simulink model "Induction_machine_qd0model_Turr"  (R2021b)
settings: Solver=FixedStepDiscrete  StartTime=0.0  StopTime=10  FixedStep=Ts  RelTol=1e-3
InitFcn:
  | Ts=1e-5;
  | fe=50;
  | Vrms=230;
undefined symbols (not defined in the file): DiscIntNeverNeededParam
settings Model: Creator=tturr  LastModifiedBy=lecci

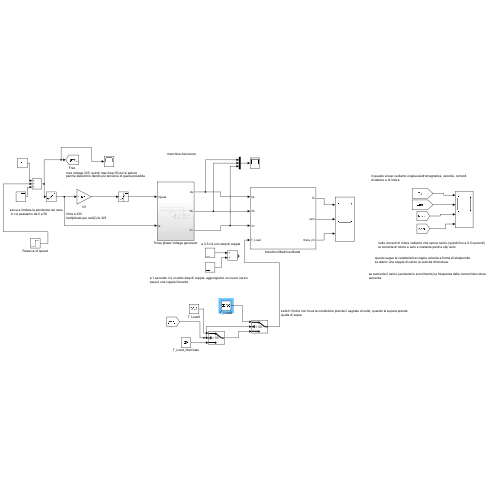
[thumbnail: Simulink's stored preview of the top-level diagram]
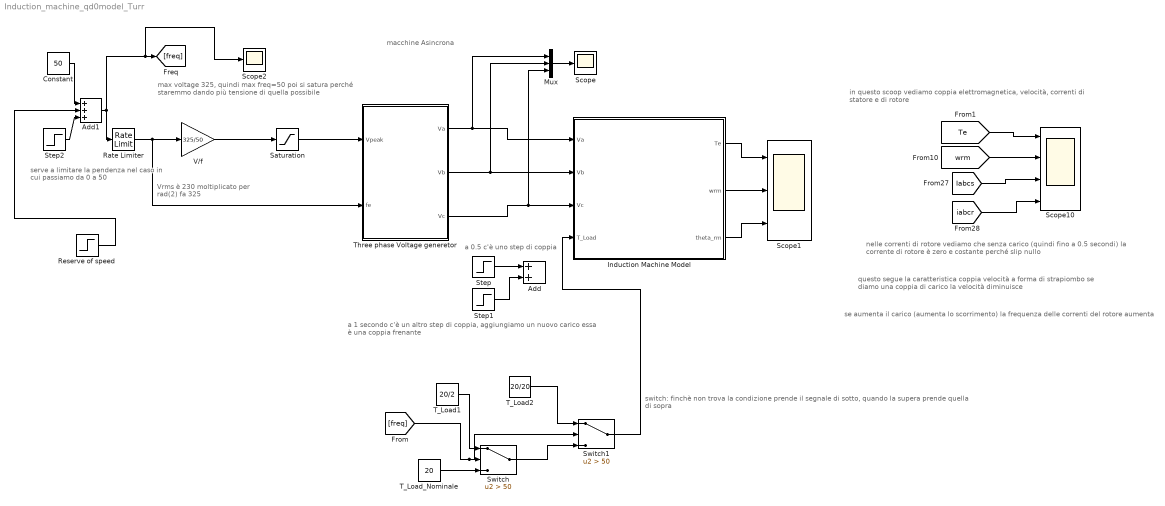
== system Induction_machine_qd0model_Turr ==
  note: switch: finchè non trova la condizione prende il segnale di sotto, quando la supera prende quella di sopra
  note: serve a limitare la pendenza nel caso
      |  in cui passiamo da 0 a 50
  note: max voltage 325, quindi max freq=50 poi si satura
      | perché staremmo dando più tensione di quella possibile
  note: Vrms è 230
      | moltiplicato per rad(2) fa 325
  note: se aumenta il carico (aumenta lo scorrimento) la frequenza delle correnti del rotore aumenta
  note: questo segue la caratteristica coppia velocità a forma di strapiombo
      | se diamo una coppia di carico la velocità diminuisce
  note: macchine Asincrona
  note: nelle correnti di rotore vediamo che senza carico (quindi fino a 0.5 secondi)
      | la corrente di rotore è zero e costante perché slip nullo
  note: in questo scoop vediamo coppia elettromagnetica, velocità, correnti
      | di statore e di rotore
  note: a 1 secondo c'è un altro step di coppia, aggiungiamo un nuovo carico
      | essa è una coppia frenante
  note: a 0.5 c'è uno step di coppia
  Add : Sum
  Add1 : Sum  Inputs=+++
  Constant : Constant  Value=50
  "Induction Machine Model " : Subsystem
  Mux : Mux  Inputs=3
  Rate Limiter : RateLimiter  RisingSlewLimit=50  FallingSlewLimit=-50  SampleTimeMode=inherited
  Reserve of speed : Step  Time=4  After=70  SampleTime=0
  Saturation : Saturate  UpperLimit=325  LowerLimit=-325
  Scope : Scope
  Scope1 : Scope  NumInputPorts=3
  Scope10 : Scope  NumInputPorts=4
  Scope2 : Scope
  Step : Step  Time=0.5  After=20  SampleTime=0
  Step1 : Step  After=20  SampleTime=0
  Step2 : Step  Time=2  After=50  SampleTime=0
  Switch : Switch  Criteria=u2 > Threshold  Threshold=50
  Switch1 : Switch  Criteria=u2 > Threshold  Threshold=50
  T_Load1 : Constant  Value=20/2
  T_Load2 : Constant  Value=20/20
  T_Load_Nominale : Constant  Value=20
  Three phase Voltage generetor : Subsystem
  V/f : Gain  Gain=325/50
  wires:
  Saturation/1 -> Three phase Voltage generetor/1(Vpeak)
  Mux/1 -> Scope/1
  Step/1 -> Add/1
  "Induction Machine Model "/2(wrm) -> Scope1/2
  "Induction Machine Model "/1(Te) -> Scope1/1
  "Induction Machine Model "/3(theta_rm) -> Scope1/3
  [wrm] -> Scope10/2
  [Te] -> Scope10/1
  [Iabcs] -> Scope10/3
  [iabcr] -> Scope10/4
  Step1/1 -> Add/2
  Three phase Voltage generetor/3(Vc) -> Mux/3, "Induction Machine Model "/3(Vc)
  Three phase Voltage generetor/2(Vb) -> Mux/2, "Induction Machine Model "/2(Vb)
  Three phase Voltage generetor/1(Va) -> Mux/1, "Induction Machine Model "/1(Va)
  V/f/1 -> Saturation/1
  Rate Limiter/1 -> Three phase Voltage generetor/2(fe), V/f/1
  Constant/1 -> Add1/1
  Step2/1 -> Add1/3
  Add1/1 -> Scope2/1, [freq], Rate Limiter/1
  T_Load_Nominale/1 -> Switch/3
  [freq] -> Switch1/2, Switch/2
  T_Load1/1 -> Switch/1
  Reserve of speed/1 -> Add1/2
  Switch/1 -> Switch1/3
  T_Load2/1 -> Switch1/1
  Switch1/1 -> "Induction Machine Model "/4(T_Load)

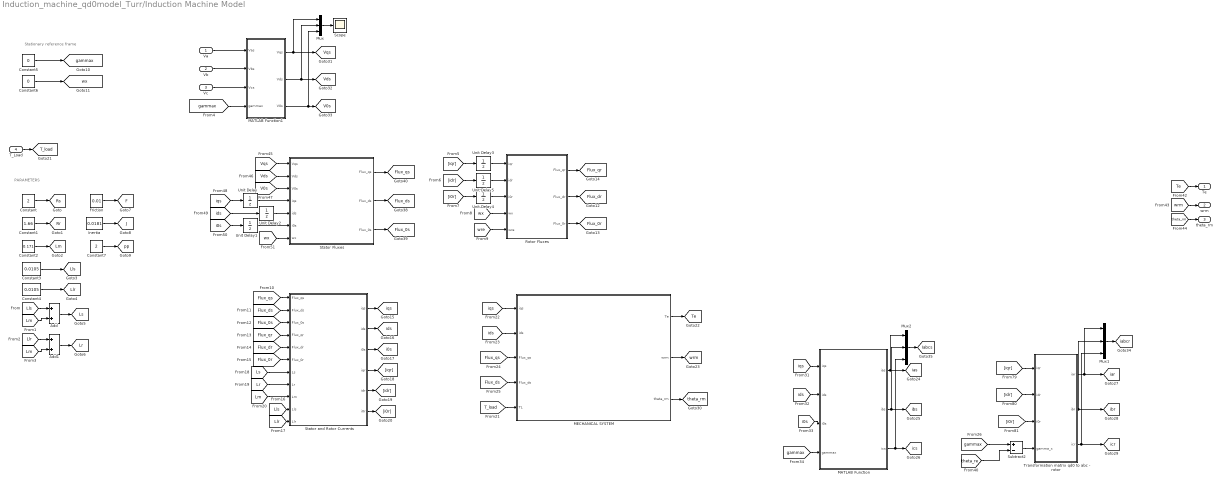
== system Induction_machine_qd0model_Turr/Induction Machine Model  ==
  note: Stationary reference frame
  note: PARAMETERS
  Va : Inport
  Vb : Inport  Port=2
  Vc : Inport  Port=3
  T_Load : Inport  Port=4
  Add : Sum
  Add1 : Sum
  Constant : Constant  Value=2
  Constant1 : Constant  Value=1.66
  Constant2 : Constant  Value=0.171
  Constant3 : Constant  Value=0.0105
  Constant4 : Constant  Value=0.0105
  Constant5 : Constant  Value=0
  Constant6 : Constant  Value=0
  Constant7 : Constant  Value=2
  Friction : Constant  Value=0.01
  Inertia : Constant  Value=0.0181
  MATLAB Function : MATLAB Function  TreatAsAtomicUnit=on
  MATLAB Function1 : MATLAB Function  TreatAsAtomicUnit=on
  MECHANICAL SYSTEM : Subsystem
  Mux : Mux  Inputs=3
  Mux1 : Mux  Inputs=3
  Mux2 : Mux  Inputs=3
  Rotor Fluxes : Subsystem
  Scope : Scope
  Stator Fluxes : Subsystem
  Stator and Rotor Currents : MATLAB Function  TreatAsAtomicUnit=on
  Subtract2 : Sum  Inputs=+-
  Transformation matrix qd0 to abc - rotor : MATLAB Function  TreatAsAtomicUnit=on
  Unit Delay{,1..5} (6 alike) : UnitDelay  SampleTime=-1  HasFrameUpgradeWarning=on
  Te : Outport
  wrm : Outport  Port=2
  theta_rm : Outport  Port=3
  tag scope: F=global, Flux_0r=global, Flux_0s=global, Flux_dr=global, Flux_ds=global, Flux_qr=global, Flux_qs=global, Iabcs=global, J=global, Llr=global, Lls=global, Lm=global, Lr=global, Ls=global, Rr=global, Rs=global, T_load=global, Te=global, V0s=global, Vds=global, Vqs=global, gammax=global, i0s=global, iabcr=global, iar=global, ias=global, ibr=global, ibs=global, icr=global, ics=global, ids=global, iqs=global, pp=global, theta_rm=global, wrm=global, wx=global
  wires:
  Constant/1 -> [Rs]
  Constant1/1 -> [Rr]
  Constant2/1 -> [Lm]
  Constant3/1 -> [Lls]
  Constant4/1 -> [Llr]
  Add/1 -> [Ls]
  [Lls] -> Add/1
  [Lm] -> Add/2
  [Lm] -> Add1/2
  [Llr] -> Add1/1
  Add1/1 -> [Lr]
  Constant7/1 -> [pp]
  Inertia/1 -> [J]
  Friction/1 -> [F]
  Va/1 -> MATLAB Function1/1(Vas)
  Vb/1 -> MATLAB Function1/2(Vbs)
  Vc/1 -> MATLAB Function1/3(Vcs)
  Constant5/1 -> [gammax]
  Constant6/1 -> [wx]
  [gammax] -> MATLAB Function1/4(gammax)
  Mux/1 -> Scope/1
  MATLAB Function1/1(Vqs) -> Mux/1, [Vqs]
  MATLAB Function1/2(Vds) -> [Vds], Mux/2
  MATLAB Function1/3(V0s) -> [V0s], Mux/3
  [Te] -> Te/1
  [wrm] -> wrm/1
  [theta_rm] -> theta_rm/1
  Stator Fluxes/1(Flux_qs) -> [Flux_qs]
  Stator Fluxes/2(Flux_ds) -> [Flux_ds]
  Stator Fluxes/3(Flux_0s) -> [Flux_0s]
  [Vqs] -> Stator Fluxes/1(Vqs)
  [Vds] -> Stator Fluxes/2(Vds)
  [V0s] -> Stator Fluxes/3(V0s)
  [ids] -> Unit Delay2/1
  [i0s] -> Unit Delay1/1
  [wx] -> Stator Fluxes/7(wx)
  [iqs] -> Unit Delay/1
  Unit Delay/1 -> Stator Fluxes/4(iqs)
  Unit Delay1/1 -> Stator Fluxes/6(i0s)
  Unit Delay2/1 -> Stator Fluxes/5(ids)
  [iqr] -> Unit Delay3/1
  [i0r] -> Unit Delay4/1
  [idr] -> Unit Delay5/1
  Unit Delay3/1 -> Rotor Fluxes/1(iqr)
  Unit Delay5/1 -> Rotor Fluxes/2(idr)
  Unit Delay4/1 -> Rotor Fluxes/3(i0r)
  [wx] -> Rotor Fluxes/4(wx)
  [wre] -> Rotor Fluxes/5(wre)
  Rotor Fluxes/1(Flux_qr) -> [Flux_qr]
  Rotor Fluxes/2(Flux_dr) -> [Flux_dr]
  Rotor Fluxes/3(Flux_0r) -> [Flux_0r]
  Stator and Rotor Currents/1(iqs) -> [iqs]
  Stator and Rotor Currents/2(ids) -> [ids]
  Stator and Rotor Currents/3(i0s) -> [i0s]
  Stator and Rotor Currents/4(iqr) -> [iqr]
  Stator and Rotor Currents/5(idr) -> [idr]
  Stator and Rotor Currents/6(i0r) -> [i0r]
  [Flux_qs] -> Stator and Rotor Currents/1(Flux_qs)
  [Flux_ds] -> Stator and Rotor Currents/2(Flux_ds)
  [Flux_0s] -> Stator and Rotor Currents/3(Flux_0s)
  [Flux_qr] -> Stator and Rotor Currents/4(Flux_qr)
  [Flux_dr] -> Stator and Rotor Currents/5(Flux_dr)
  [Flux_0r] -> Stator and Rotor Currents/6(Flux_0r)
  [Ls] -> Stator and Rotor Currents/7(Ls)
  [Lr] -> Stator and Rotor Currents/8(Lr)
  [Lm] -> Stator and Rotor Currents/9(Lm)
  [Lls] -> Stator and Rotor Currents/10(Lls)
  [Llr] -> Stator and Rotor Currents/11(Llr)
  Transformation matrix qd0 to abc - rotor/3(icr) -> Mux1/3, [icr]
  [idr] -> Transformation matrix qd0 to abc - rotor/2(idr)
  [i0r] -> Transformation matrix qd0 to abc - rotor/3(i0r)
  [ids] -> MATLAB Function/2(ids)
  MATLAB Function/3(ics) -> Mux2/3, [ics]
  Transformation matrix qd0 to abc - rotor/1(iar) -> Mux1/1, [iar]
  MATLAB Function/1(ias) -> Mux2/1, [ias]
  [theta_re] -> Subtract2/2
  [iqr] -> Transformation matrix qd0 to abc - rotor/1(iqr)
  Subtract2/1 -> Transformation matrix qd0 to abc - rotor/4(gamma_x)
  MATLAB Function/2(ibs) -> Mux2/2, [ibs]
  [gammax] -> MATLAB Function/4(gammax)
  [iqs] -> MATLAB Function/1(iqs)
  [i0s] -> MATLAB Function/3(i0s)
  [gammax] -> Subtract2/1
  T_Load/1 -> [T_load]
  [T_load] -> MECHANICAL SYSTEM/5(TL)
  [iqs] -> MECHANICAL SYSTEM/1(iqs)
  [ids] -> MECHANICAL SYSTEM/2(ids)
  [Flux_ds] -> MECHANICAL SYSTEM/4(Flux_ds)
  [Flux_qs] -> MECHANICAL SYSTEM/3(Flux_qs)
  MECHANICAL SYSTEM/1(Te) -> [Te]
  MECHANICAL SYSTEM/2(wrm) -> [wrm]
  MECHANICAL SYSTEM/3(theta_rm) -> [theta_rm]
  Transformation matrix qd0 to abc - rotor/2(ibr) -> Mux1/2, [ibr]
  Mux1/1 -> [iabcr]
  Mux2/1 -> [Iabcs]

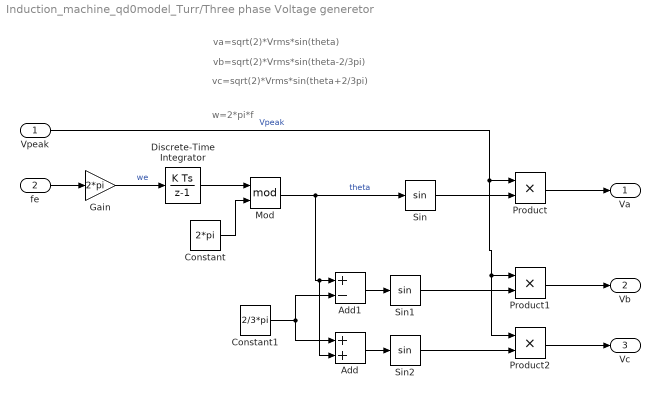
== system Induction_machine_qd0model_Turr/Three phase Voltage generetor ==
  note: w=2*pi*f
  note: va=sqrt(2)*Vrms*sin(theta)
  note: vb=sqrt(2)*Vrms*sin(theta-2/3pi)
  note: vc=sqrt(2)*Vrms*sin(theta+2/3pi)
  Vpeak : Inport
  fe : Inport  Port=2
  Add : Sum
  Add1 : Sum  Inputs=+-
  Constant : Constant  Value=2*pi
  Constant1 : Constant  Value=2/3*pi
  Discrete-Time Integrator : DiscreteIntegrator  SampleTime=-1  ICPrevOutput=DiscIntNeverNeededParam  ICPrevScaledInput=DiscIntNeverNeededParam
  Gain : Gain  Gain=2*pi
  Mod : Math  Operator=mod  SaturateOnIntegerOverflow=on
  Product : Product
  Product1 : Product
  Product2 : Product
  Sin : Trigonometry
  Sin1 : Trigonometry
  Sin2 : Trigonometry
  Va : Outport
  Vb : Outport  Port=2
  Vc : Outport  Port=3
  wires:
  fe/1 -> Gain/1
  Gain/1 -> Discrete-Time Integrator/1  "we"
  Discrete-Time Integrator/1 -> Mod/1
  Constant/1 -> Mod/2
  Mod/1 -> Add/2, Add1/1, Sin/1  "theta"
  Vpeak/1 -> Product2/1, Product1/1, Product/1  "Vpeak"
  Sin/1 -> Product/2
  Product/1 -> Va/1
  Product1/1 -> Vb/1
  Sin1/1 -> Product1/2
  Sin2/1 -> Product2/2
  Product2/1 -> Vc/1
  Constant1/1 -> Add1/2, Add/1
  Add1/1 -> Sin1/1
  Add/1 -> Sin2/1

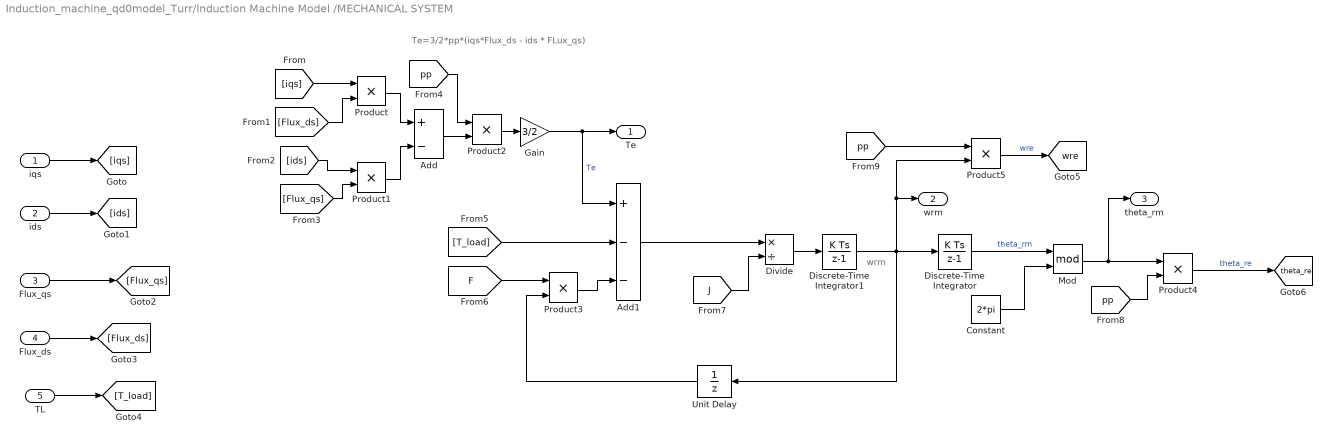
== system Induction_machine_qd0model_Turr/Induction Machine Model /MECHANICAL SYSTEM ==
  note: wrm
  note: Te=3/2*pp*(iqs*Flux_ds - ids * FLux_qs)
  iqs : Inport
  ids : Inport  Port=2
  Flux_qs : Inport  Port=3
  Flux_ds : Inport  Port=4
  TL : Inport  Port=5
  Add : Sum  Inputs=+-
  Add1 : Sum  Inputs=+--
  Constant : Constant  Value=2*pi
  Discrete-Time Integrator : DiscreteIntegrator  SampleTime=-1  ICPrevOutput=DiscIntNeverNeededParam  ICPrevScaledInput=DiscIntNeverNeededParam
  Discrete-Time Integrator1 : DiscreteIntegrator  SampleTime=-1  ICPrevOutput=DiscIntNeverNeededParam  ICPrevScaledInput=DiscIntNeverNeededParam
  Divide : Product  Inputs=*/
  Gain : Gain  Gain=3/2
  Mod : Math  Operator=mod  SaturateOnIntegerOverflow=on
  Product{,1..5} (6 alike) : Product
  Unit Delay : UnitDelay  SampleTime=-1  HasFrameUpgradeWarning=on
  Te : Outport
  wrm : Outport  Port=2
  theta_rm : Outport  Port=3
  tag scope: theta_re=global, wre=global
  wires:
  iqs/1 -> [iqs]
  ids/1 -> [ids]
  Flux_qs/1 -> [Flux_qs]
  Flux_ds/1 -> [Flux_ds]
  [iqs] -> Product/1
  [Flux_ds] -> Product/2
  Product/1 -> Add/1
  [ids] -> Product1/1
  [Flux_qs] -> Product1/2
  Product1/1 -> Add/2
  Product2/1 -> Gain/1
  Add/1 -> Product2/2
  [pp] -> Product2/1
  Gain/1 -> Add1/1, Te/1  "Te"
  TL/1 -> [T_load]
  [T_load] -> Add1/2
  Product3/1 -> Add1/3
  [F] -> Product3/1
  Add1/1 -> Divide/1
  [J] -> Divide/2
  Divide/1 -> Discrete-Time Integrator1/1
  Unit Delay/1 -> Product3/2
  Discrete-Time Integrator1/1 -> wrm/1, Product5/2, Discrete-Time Integrator/1, Unit Delay/1
  Discrete-Time Integrator/1 -> Mod/1  "theta_rm"
  Constant/1 -> Mod/2
  Mod/1 -> theta_rm/1, Product4/1
  [pp] -> Product4/2
  Product4/1 -> [theta_re]  "theta_re"
  [pp] -> Product5/1
  Product5/1 -> [wre]  "wre"

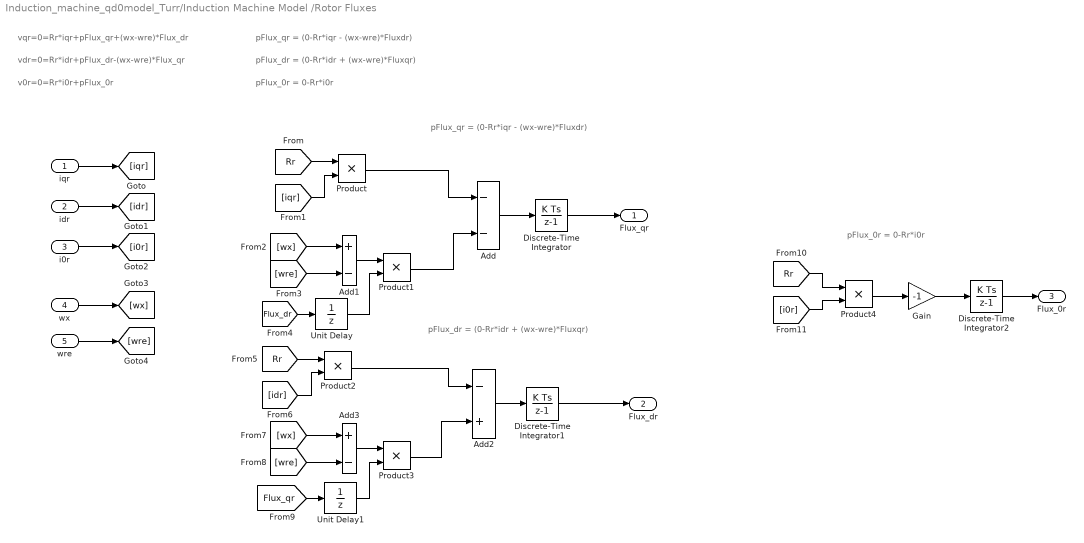
== system Induction_machine_qd0model_Turr/Induction Machine Model /Rotor Fluxes ==
  note: vdr=0=Rr*idr+pFlux_dr-(wx-wre)*Flux_qr
  note: v0r=0=Rr*i0r+pFlux_0r
  note: vqr=0=Rr*iqr+pFlux_qr+(wx-wre)*Flux_dr
  note: pFlux_qr = (0-Rr*iqr - (wx-wre)*Fluxdr)
  note: pFlux_dr = (0-Rr*idr + (wx-wre)*Fluxqr)
  note: pFlux_0r = 0-Rr*i0r
  note: pFlux_qr = (0-Rr*iqr - (wx-wre)*Fluxdr)
  note: pFlux_dr = (0-Rr*idr + (wx-wre)*Fluxqr)
  note: pFlux_0r = 0-Rr*i0r
  iqr : Inport
  idr : Inport  Port=2
  i0r : Inport  Port=3
  wx : Inport  Port=4
  wre : Inport  Port=5
  Add : Sum  Inputs=--
  Add1 : Sum  Inputs=+-
  Add2 : Sum  Inputs=-+
  Add3 : Sum  Inputs=+-
  Discrete-Time Integrator : DiscreteIntegrator  SampleTime=-1  ICPrevOutput=DiscIntNeverNeededParam  ICPrevScaledInput=DiscIntNeverNeededParam
  Discrete-Time Integrator1 : DiscreteIntegrator  SampleTime=-1  ICPrevOutput=DiscIntNeverNeededParam  ICPrevScaledInput=DiscIntNeverNeededParam
  Discrete-Time Integrator2 : DiscreteIntegrator  SampleTime=-1  ICPrevOutput=DiscIntNeverNeededParam  ICPrevScaledInput=DiscIntNeverNeededParam
  Gain : Gain  Gain=-1
  Product{,1..4} (5 alike) : Product
  Unit Delay : UnitDelay  SampleTime=-1  HasFrameUpgradeWarning=on
  Unit Delay1 : UnitDelay  SampleTime=-1  HasFrameUpgradeWarning=on
  Flux_qr : Outport
  Flux_dr : Outport  Port=2
  Flux_0r : Outport  Port=3
  wires:
  iqr/1 -> [iqr]
  i0r/1 -> [i0r]
  idr/1 -> [idr]
  wx/1 -> [wx]
  wre/1 -> [wre]
  [Rr] -> Product/1
  [iqr] -> Product/2
  Product/1 -> Add/1
  [wx] -> Add1/1
  [wre] -> Add1/2
  Add1/1 -> Product1/1
  [Flux_dr] -> Unit Delay/1
  Product1/1 -> Add/2
  Add/1 -> Discrete-Time Integrator/1
  Discrete-Time Integrator/1 -> Flux_qr/1
  Product2/1 -> Add2/1
  [idr] -> Product2/2
  [Rr] -> Product2/1
  [Flux_qr] -> Unit Delay1/1
  Add3/1 -> Product3/1
  [wre] -> Add3/2
  [wx] -> Add3/1
  Product3/1 -> Add2/2
  Add2/1 -> Discrete-Time Integrator1/1
  Discrete-Time Integrator1/1 -> Flux_dr/1
  Product4/1 -> Gain/1
  [Rr] -> Product4/1
  [i0r] -> Product4/2
  Gain/1 -> Discrete-Time Integrator2/1
  Discrete-Time Integrator2/1 -> Flux_0r/1
  Unit Delay/1 -> Product1/2
  Unit Delay1/1 -> Product3/2

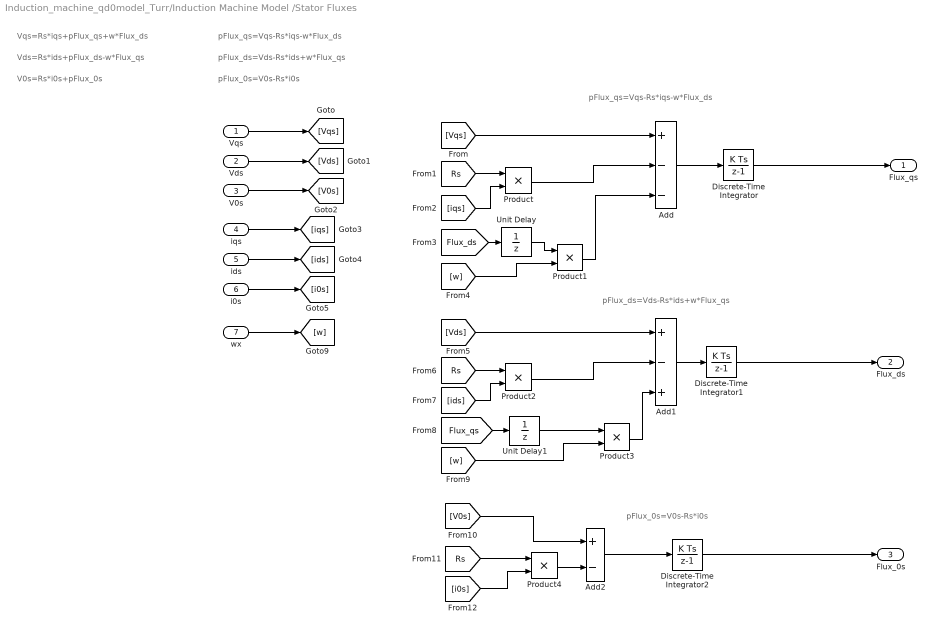
== system Induction_machine_qd0model_Turr/Induction Machine Model /Stator Fluxes ==
  note: Vqs=Rs*iqs+pFlux_qs+w*Flux_ds
  note: Vds=Rs*ids+pFlux_ds-w*Flux_qs
  note: V0s=Rs*i0s+pFlux_0s
  note: pFlux_qs=Vqs-Rs*iqs-w*Flux_ds
  note: pFlux_ds=Vds-Rs*ids+w*Flux_qs
  note: pFlux_0s=V0s-Rs*i0s
  note: pFlux_0s=V0s-Rs*i0s
  note: pFlux_ds=Vds-Rs*ids+w*Flux_qs
  note: pFlux_qs=Vqs-Rs*iqs-w*Flux_ds
  Vqs : Inport
  Vds : Inport  Port=2
  V0s : Inport  Port=3
  iqs : Inport  Port=4
  ids : Inport  Port=5
  i0s : Inport  Port=6
  wx : Inport  Port=7
  Add : Sum  Inputs=+--
  Add1 : Sum  Inputs=+-+
  Add2 : Sum  Inputs=+-
  Discrete-Time Integrator : DiscreteIntegrator  SampleTime=-1  ICPrevOutput=DiscIntNeverNeededParam  ICPrevScaledInput=DiscIntNeverNeededParam
  Discrete-Time Integrator1 : DiscreteIntegrator  SampleTime=-1  ICPrevOutput=DiscIntNeverNeededParam  ICPrevScaledInput=DiscIntNeverNeededParam
  Discrete-Time Integrator2 : DiscreteIntegrator  SampleTime=-1  ICPrevOutput=DiscIntNeverNeededParam  ICPrevScaledInput=DiscIntNeverNeededParam
  Product{,1..4} (5 alike) : Product
  Unit Delay : UnitDelay  SampleTime=-1  HasFrameUpgradeWarning=on
  Unit Delay1 : UnitDelay  SampleTime=-1  HasFrameUpgradeWarning=on
  Flux_qs : Outport
  Flux_ds : Outport  Port=2
  Flux_0s : Outport  Port=3
  wires:
  Vqs/1 -> [Vqs]
  Vds/1 -> [Vds]
  V0s/1 -> [V0s]
  iqs/1 -> [iqs]
  ids/1 -> [ids]
  i0s/1 -> [i0s]
  [Vqs] -> Add/1
  [Rs] -> Product/1
  [iqs] -> Product/2
  Product/1 -> Add/2
  [Flux_ds] -> Unit Delay/1
  wx/1 -> [w]
  [w] -> Product1/2
  Product1/1 -> Add/3
  Unit Delay/1 -> Product1/1
  Add/1 -> Discrete-Time Integrator/1
  Discrete-Time Integrator/1 -> Flux_qs/1
  [Vds] -> Add1/1
  [Rs] -> Product2/1
  Product2/1 -> Add1/2
  [ids] -> Product2/2
  Unit Delay1/1 -> Product3/1
  [w] -> Product3/2
  Product3/1 -> Add1/3
  [Flux_qs] -> Unit Delay1/1
  Add1/1 -> Discrete-Time Integrator1/1
  Discrete-Time Integrator1/1 -> Flux_ds/1
  [i0s] -> Product4/2
  [Rs] -> Product4/1
  Product4/1 -> Add2/2
  [V0s] -> Add2/1
  Add2/1 -> Discrete-Time Integrator2/1
  Discrete-Time Integrator2/1 -> Flux_0s/1

== matlab function Induction_machine_qd0model_Turr/Induction Machine Model /MATLAB Function1 ==
  data: Vas input; Vqs output; Vbs input; Vcs input; gammax input; Vds output; V0s output
function [Vqs, Vds, V0s] = fcn(Vas, Vbs, Vcs, gammax)

Vabcs=[Vas; Vbs; Vcs];

K=2/3*[cos(gammax)    cos(gammax-2/3*pi)  cos(gammax+2/3*pi);
       sin(gammax)    sin(gammax-2/3*pi)  sin(gammax+2/3*pi); ...
        1/2  1/2  1/2];

Vqds=K*Vabcs;

Vqs=Vqds(1);
Vds=Vqds(2);
V0s=Vqds(3);

== matlab function Induction_machine_qd0model_Turr/Induction Machine Model /Stator and Rotor Currents ==
  data: Flux_qs input; iqs output; Flux_ds input; Flux_0s input; Flux_qr input; Flux_dr input; Flux_0r input; Ls input; Lr input; Lm input; Lls input; ids output; i0s output; iqr output; idr output; i0r output; Llr input
function [iqs, ids, i0s, iqr, idr, i0r] = fcn(Flux_qs, Flux_ds, Flux_0s, Flux_qr, Flux_dr, Flux_0r, Ls,Lr,Lm, Lls, Llr)

Flux=[Flux_qs; Flux_ds; Flux_qr; Flux_dr];

L=[Ls 0 Lm 0;
   0 Ls 0 Lm;
   Lm 0 Lr 0;
   0 Lm 0 Lr];

iqd=inv(L)*Flux;

iqs=iqd(1);
ids=iqd(2);
iqr=iqd(3);
idr=iqd(4);

i0s=Flux_0s/Lls;
i0r=Flux_0r/Llr;

== matlab function Induction_machine_qd0model_Turr/Induction Machine Model /MATLAB Function ==
  data: iqs input; ias output; ids input; i0s input; gammax input; ibs output; ics output
function [ias,ibs,ics] = fcn(iqs,ids,i0s,gammax)

Iqd0s=[iqs ids i0s]';
invK=[cos(gammax) sin(gammax) 1;
    cos(gammax-2/3*pi) sin(gammax-2/3*pi) 1;
    cos(gammax+2/3*pi) sin(gammax+2/3*pi) 1];
Iabcs=invK*Iqd0s;
ias=Iabcs(1);
ibs=Iabcs(2);
ics=Iabcs(3);

== matlab function Induction_machine_qd0model_Turr/Induction Machine Model /Transformation matrix qd0 to abc - rotor ==
  data: iqr input; iar output; idr input; i0r input; gamma_x input; ibr output; icr output
function [iar, ibr, icr] = fcn(iqr, idr, i0r, gamma_x)

Iqd0r = [iqr;idr;i0r];

invK = [cos(gamma_x) sin(gamma_x) 1;
    cos(gamma_x-2/3*pi) sin(gamma_x-2/3*pi) 1;
    cos(gamma_x+2/3*pi) sin(gamma_x+2/3*pi) 1];

Iabcr = invK*Iqd0r;

iar = Iabcr(1);
ibr = Iabcr(2);
icr = Iabcr(3);
